simulink model "model_problem4"  (R2020a)
settings: Solver=VariableStepAuto  StartTime=0.0  StopTime=10.0  RelTol=1e-3
values from neighbouring files (symbols this model uses):
  b = 3.5077E-66    (= 3.5077e-66)    [initialisation.m]
  J = 3.2284E-6    (= 3.2284e-06)    [initialisation.m]
  ke = 0.0274    [initialisation.m]
  kt = 0.0274    [initialisation.m]
  L = 2.75E-6    (= 2.75e-06)    [initialisation.m]
  R = 4    [initialisation.m]
libraries: simulink x1
settings Model: Creator=Prateek  LastModifiedBy=Prateek

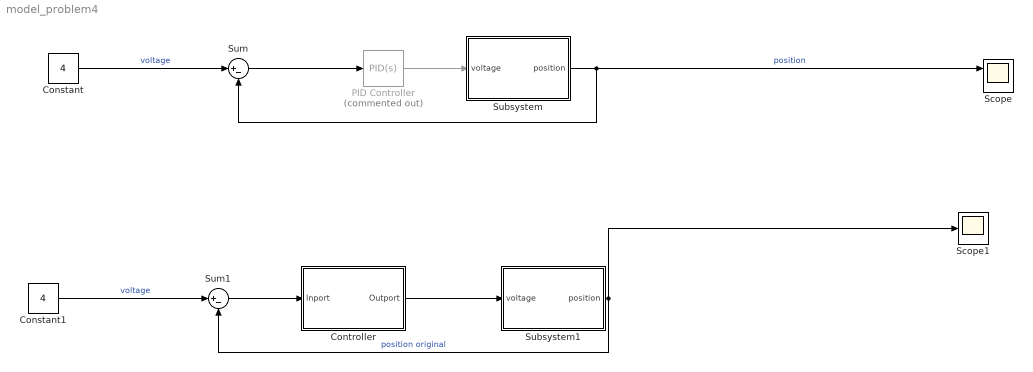
== system model_problem4 ==
  Constant : Constant  Value=4
  Constant1 : Constant  Value=4
  Controller : Subsystem
  PID Controller : simulink/Continuous/PID Controller  Commented=on  Controller=PID  Form=Parallel  TimeDomain=Continuous-time  UseExternalTs=off  SampleTime=-1  IntegratorMethod=Forward Euler  FilterMethod=Forward Euler  ControllerParametersSource=internal  P=1  I=1  D=0  UseFilter=on  N=1  TunerSelectOption=Transfer Function Based (PID Tuner App)  InitialConditionSource=internal  InitialConditionForIntegrator=0  InitialConditionForFilter=0  DifferentiatorICPrevScaledInput=0  ExternalReset=none  TrackingMode=off  Kt=1  LimitOutput=off  UpperSaturationLimit=inf  LowerSaturationLimit=-inf  LinearizeAsGain=on  AntiWindupMode=none  Kb=1  POutMin=[]  POutMax=[]  IOutMin=[]  IOutMax=[]  DOutMin=[]  DOutMax=[]  NOutMin=[]  NOutMax=[]  SumOutMin=[]  SumOutMax=[]  SaturationOutMin=[]  SaturationOutMax=[]  PParamMin=[]  PParamMax=[]  IParamMin=[]  IParamMax=[]  DParamMin=[]  DParamMax=[]  NParamMin=[]  NParamMax=[]  KbParamMin=[]  KbParamMax=[]  KtParamMin=[]  KtParamMax=[]  KbOutMin=[]  KbOutMax=[]  KtOutMin=[]  KtOutMax=[]  IntegratorOutMin=[]  IntegratorOutMax=[]  FilterOutMin=[]  FilterOutMax=[]  SumI1OutMin=[]  SumI1OutMax=[]  SumI2OutMin=[]  SumI2OutMax=[]  SumI3OutMin=[]  SumI3OutMax=[]  SumI4OutMin=[]  SumI4OutMax=[]  SumDOutMin=[]  SumDOutMax=[]  DifferentiatorOutMin=[]  DifferentiatorOutMax=[]  FilterDiffOutCoefMin=[]  FilterDiffOutCoefMax=[]  ReciprocalOutMin=[]  ReciprocalOutMax=[]  SumDenOutMin=[]  SumDenOutMax=[]  SumNumOutMin=[]  SumNumOutMax=[]  DivideOutMin=[]  DivideOutMax=[]  UdiffTsProdOutMin=[]  UdiffTsProdOutMax=[]  NTsProdOutMin=[]  NTsProdOutMax=[]  UintegralTsProdOutMin=[]  UintegralTsProdOutMax=[]  UngainTsProdOutMin=[]  UngainTsProdOutMax=[]  IntegratorContinuousStateAttributes=''  IntegratorStateMustResolveToSignalObject=off  IntegratorRTWStateStorageClass=Auto  FilterContinuousStateAttributes=''  FilterStateMustResolveToSignalObject=off  FilterRTWStateStorageClass=Auto  ParallelPVariant=InternalParameters  IdealPVariant=Disabled  IVariant=InternalParameters  DVariant=InternalParameters  IntegratorVariant=Continuous  SatVariant=Disabled  AWVariant=Passthrough  PCopyVariant=Disabled  TRVariant=Disabled  FdbkBlocksVariant=Forward  IdealPFdbkVariant=Disabled  SatFdbkVariant=Disabled  DerivativeFilterVariant=ContFilter  NVariant=InternalParameters  NCopyVariant=Disabled  FilterICVariant=InternalICsFilter  IntegratorICVariant=InternalICs  ExternalResetVariant=Disabled  TRSumVariant=Passthrough  SumFdbkVariant=Disabled  SumVariant=Sum_PID  TsampFilterVariant=InternalTs  TsampNgainVariant=Passthrough  TsampIntegralVariant=Passthrough
  Scope : Scope  NumInputPorts=2
  Scope1 : Scope
  Subsystem : Subsystem
  Subsystem1 : Subsystem
  Sum : Sum  Inputs=|+-
  Sum1 : Sum  Inputs=|+-
  wires:
  Subsystem/1(position) -> Scope/1, Sum/2  "position"
  Constant/1 -> Sum/1  "voltage"
  PID Controller/1 -> Subsystem/1(voltage)
  Sum/1 -> PID Controller/1
  Controller/1(Outport) -> Subsystem1/1(voltage)
  Constant1/1 -> Sum1/1  "voltage"
  Subsystem1/1(position) -> Scope1/1, Sum1/2  "position original"
  Sum1/1 -> Controller/1(Inport)

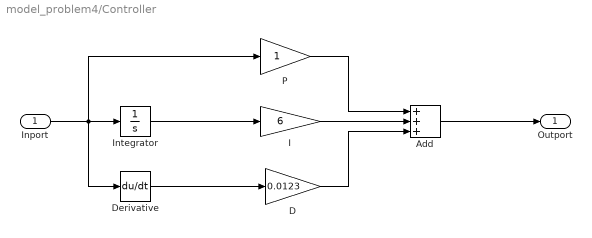
== system model_problem4/Controller ==
  Inport : Inport
  Add : Sum  Inputs=+++
  D : Gain  Gain=0.0123
  Derivative : Derivative
  I : Gain  Gain=6
  Integrator : Integrator
  P : Gain
  Outport : Outport
  wires:
  Inport/1 -> P/1, Integrator/1, Derivative/1
  D/1 -> Add/3
  P/1 -> Add/1
  I/1 -> Add/2
  Add/1 -> Outport/1
  Integrator/1 -> I/1
  Derivative/1 -> D/1

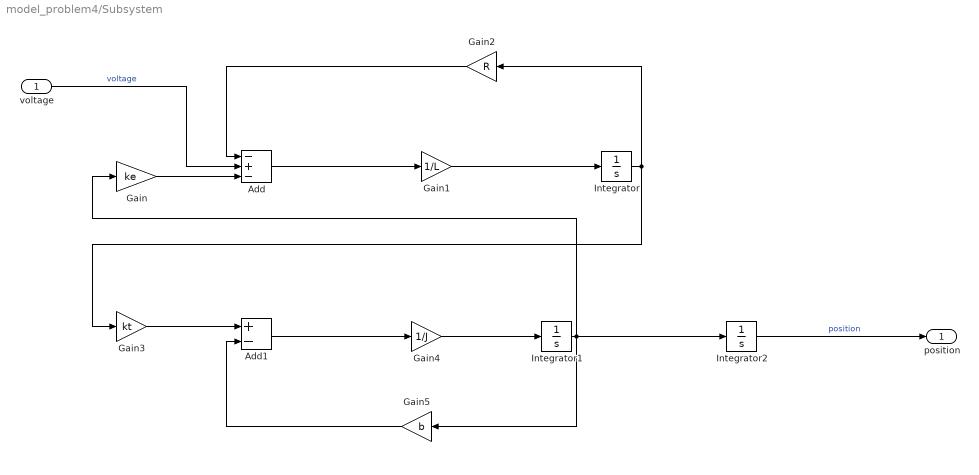
== system model_problem4/Subsystem ==
  voltage : Inport
  Add : Sum  Inputs=-+-
  Add1 : Sum  Inputs=+-
  Gain : Gain  Gain=ke
  Gain1 : Gain  Gain=1/L
  Gain2 : Gain  Gain=R
  Gain3 : Gain  Gain=kt
  Gain4 : Gain  Gain=1/J
  Gain5 : Gain  Gain=b
  Integrator : Integrator
  Integrator1 : Integrator
  Integrator2 : Integrator
  position : Outport
  wires:
  Gain1/1 -> Integrator/1
  Add1/1 -> Gain4/1
  Integrator/1 -> Gain3/1, Gain2/1
  Add/1 -> Gain1/1
  Integrator1/1 -> Gain/1, Integrator2/1, Gain5/1
  Integrator2/1 -> position/1  "position"
  Gain2/1 -> Add/1
  voltage/1 -> Add/2  "voltage"
  Gain/1 -> Add/3
  Gain3/1 -> Add1/1
  Gain4/1 -> Integrator1/1
  Gain5/1 -> Add1/2

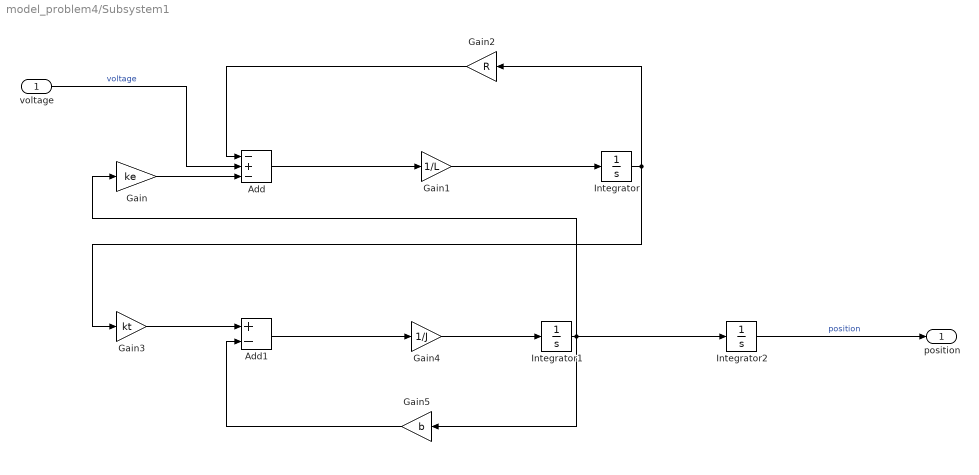
== system model_problem4/Subsystem1 ==
  voltage : Inport
  Add : Sum  Inputs=-+-
  Add1 : Sum  Inputs=+-
  Gain : Gain  Gain=ke
  Gain1 : Gain  Gain=1/L
  Gain2 : Gain  Gain=R
  Gain3 : Gain  Gain=kt
  Gain4 : Gain  Gain=1/J
  Gain5 : Gain  Gain=b
  Integrator : Integrator
  Integrator1 : Integrator
  Integrator2 : Integrator
  position : Outport
  wires:
  Gain1/1 -> Integrator/1
  Add1/1 -> Gain4/1
  Integrator/1 -> Gain3/1, Gain2/1
  Add/1 -> Gain1/1
  Integrator1/1 -> Gain/1, Integrator2/1, Gain5/1
  Integrator2/1 -> position/1  "position"
  Gain2/1 -> Add/1
  voltage/1 -> Add/2  "voltage"
  Gain/1 -> Add/3
  Gain3/1 -> Add1/1
  Gain4/1 -> Integrator1/1
  Gain5/1 -> Add1/2
